simulink model "twin_sldemo_autotrans_old"  (Simulink 9.0)
settings: Solver=ode5  StartTime=0.0  StopTime=150.0  RelTol=1e-3  AbsTol=1e-6
model workspace (MAT data in the model file):
  CONVERTER_DATA = [0  137.465208994  2.232; 0.1  137.065019157  2.075; 0.2  135.864449646  1.975; 0.3  135.664354728  1.846; 0.4  137.565256453  1.72; 0.5  140.366585312  1.564; 0.6  145.268910814  1.409; 0.7  152.872517717  1.254; 0.8  162.9773111  1.096; 0.81  164.27792807  1.08; 0.82  166.178829795  1.061; 0.83  167.979684062  1.043; 0.84  170.080680706  1.028; 0.85  172.781962105  1.012; 0.86  175.383196045  1.002; 0.87  179.585189333  1.002; 0.88  183.587087703  1.001; 0.89  189.890077635  0.998; 0.9  197.693779455  0.999; 0.92  215.902417037  1.001; 0.94  244.515990379  1.002]
  DOWN_TABLE = [0  5  20  35; 0  5  20  35; 0  5  25  40; 0  5  30  50; 0  30  50  80; 0  30  50  80]
  DOWN_TH_BP = [0; 5; 40; 50; 90; 100]
  EMAP = [-40  -44  -49  -53  -57  -61  -65  -70  -74  -78  -82; 215  117  85  66  44  29  10  -2  -13  -22  -32; 245  208  178  148  122  104  85  66  48  33  18; 264  260  241  219  193  167  152  133  119  96  85; 264  279  282  275  260  238  223  208  189  171  152; 267  290  293  297  290  275  260  256  234  212  193; 267  297  305  305  305  301  293  282  267  249  226; 267  301  308  312  319  323  319  316  297  279  253; 267  301  312  319  327  327  327  327  312  293  267; 267  301  312  319  327  334  334  334  319  305  275]
  Iei = 0.0219914882836
  NE_VEC = [800 1200 1600 2000 2400 2800 3200 3600 4000 4400 4800]
  TH_VEC = [0; 20; 30; 40; 50; 60; 70; 80; 90; 100]
  TWAIT = 2
  UP_TABLE = [10  30  50  1000000; 10  30  50  1000000; 15  30  50  1000000; 23  41  60  1000000; 40  70  100  1000000; 40  70  100  1000000]
  UP_TH_BP = [0; 25; 35; 50; 90; 100]
  VEHICLE_DATA : num (value not decoded)
undefined symbols (not defined in the file or in its folder): sigbuilder_block
Description:
  | Modeling an Automatic Transmission Controller
  | 
  | In this example, Simulink(R) is used to model an automotive drivetrain. Stateflow(R)
  | enhances the Simulink model with its representation of the transmission
  | control logic. Simulink provides a powerful environment for the modeling and
  | simulation of dynamic systems and processes. In many systems, though,
  | supervisory functions like changing modes or invoking new gain schedules must
  | respond to events that may occur and conditions that develop over time. As a
  | result, the environment requires a language capable of managing these multiple
  | modes and developing conditions. In the following example, Stateflow
  | demonstrates its strength in this capacity by performing the function of gear
  | selection in an automatic transmission. This function is combined with the
  | drivetrain dynamics in a natural and intuitive manner by incorporating a
  | Stateflow block in the Simulink block diagram.
settings Model: SuppressorTable=22 serialization::archive 11 0 6 0 0 0 1 0  DataTypeOverride=Double  MinMaxOverflowLogging=ForceOff  FPTRunName=Active  Creator=The MathWorks, Inc.  LastModifiedBy=luigi  ExtModeTrigMode=oneshot  ExtModeArmWhenConnect=off  ExtModeAutoUpdateStatusClock=off
settings DataIOCC: SaveFormat=StructureWithTime  SaveOutput=off  SaveTime=off  SignalLoggingName=sldemo_autotrans_output
settings OptimizationCC: BlockReduction=off  ExpressionDepthLimit=2147483647  InitFltsAndDblsToZero=on
settings DebuggingCC: SignalInfNanChecking=error  SaveWithParameterizedLinksMsg=none  UnderspecifiedInitializationDetection=Simplified  MergeDetectMultiDrivingBlocksExec=error  CheckExecutionContextPreStartOutputMsg=on  CheckExecutionContextRuntimeOutputMsg=on  MultiTaskCondExecSysMsg=none  SigSpecEnsureSampleTimeMsg=none  IntegerOverflowMsg=none  FcnCallInpInsideContextMsg=warning  SignalLabelMismatchMsg=error  UnconnectedInputMsg=error  UnconnectedOutputMsg=error  UnconnectedLineMsg=error  UniqueDataStoreMsg=error  BusObjectLabelMismatch=error  RootOutportRequireBusObject=error  StateNameClashWarn=warning  StrictBusMsg=ErrorOnBusTreatedAsVector  NonBusSignalsTreatedAsBus=error  IntegerSaturationMsg=none
settings HardwareCC: ProdIntDivRoundTo=Floor
settings SFSimCC: SFSimEcho=off  SimParseCustomCode=off
settings GRTTargetCC: TargetFcnLib=ansi_tfl_tmw.mat  GeneratePreprocessorConditionals=Disable all  CombineOutputUpdateFcns=off  GRTInterface=on
settings ConfigComp: CovMetricSettings=dcmtr  CovHTMLOptions=-aTS=1 -bRG=1 -bTC=1 -hTR=0 -nFC=0 -scm=1 -bcm=1 -xEv=0  CovHtmlReporting=off

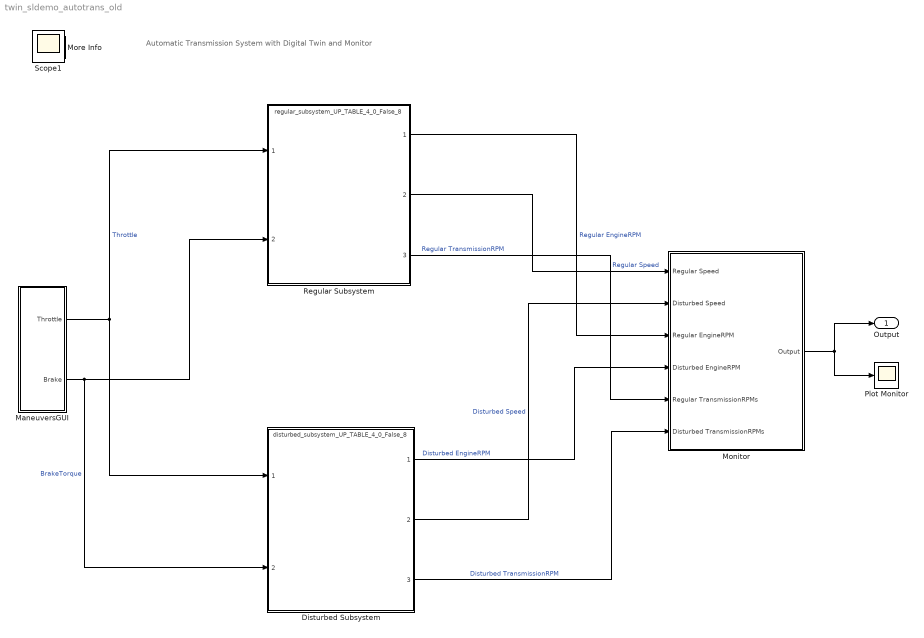
== system twin_sldemo_autotrans_old ==
  note: Automatic Transmission System with Digital Twin and Monitor
  Disturbed Subsystem : ModelReference  ModelNameDialog=disturbed_subsystem_UP_TABLE_4_0_False_8.mdl  SimulationMode=Normal  ModelReferenceVersion=1.265
  ManeuversGUI : Subsystem  Tag=STV Subsys  LoadFcn=sigbuilder_block('load');  StartFcn=sigbuilder_block('start');  StopFcn=sigbuilder_block('stop');  ClipboardFcn=sigbuilder_block('clipboard');  mask(Sigbuilder block){tuvar=[0:10]}
      mask help: Sigbuilder GUI
      mask init:
      | tuvar = sigbuilder_block('maskInit');
      settings: CopyFcn=sigbuilder_block('copy');  DeleteFcn=sigbuilder_block('delete');  ModelCloseFcn=sigbuilder_block('modelClose');  PreSaveFcn=sigbuilder_block('preSave');  PauseFcn=sigbuilder_block('pause')  ContinueFcn=sigbuilder_block('continue')  NameChangeFcn=sigbuilder_block('namechange');  OpenFcn=sigbuilder_block('open',[50.25 0 1389.75 726 ]);  CloseFcn=sigbuilder_block('close');
      mask Display: plot(0, 0, 100, 100,[2, 2, 32, 32, 2], [68, 8, 8, 68, 68],[32, 2], [38, 38], [32, 19, 2],[53, 60, 44], [32, 17, 17, 2],[16, 16, 31, 31]);txt = getActiveGroup(gcbh);text(2, 100, txt,'verticalAlignment', 'top');
  Monitor : Subsystem
  More Info : Subsystem
      settings: OpenFcn=showdemo(bdroot(gcb))
      mask Display: disp('?')
  Plot Monitor : Scope
  Regular Subsystem : ModelReference  ModelNameDialog=regular_subsystem_UP_TABLE_4_0_False_8.mdl  SimulationMode=Normal  ModelReferenceVersion=1.263
  Output : Outport
  Scope1 : Scope
  wires:
  Disturbed Subsystem/2 -> Monitor/2(Disturbed Speed)  "Disturbed Speed"
  ManeuversGUI/1(Throttle) -> Disturbed Subsystem/1, Regular Subsystem/1  "Throttle"
  Disturbed Subsystem/3 -> Monitor/6(Disturbed TransmissionRPMs)  "Disturbed TransmissionRPM"
  ManeuversGUI/2(Brake) -> Disturbed Subsystem/2, Regular Subsystem/2  "BrakeTorque"
  Monitor/1(Output) -> Plot Monitor/1, Output/1
  Regular Subsystem/1 -> Monitor/3(Regular EngineRPM)  "Regular EngineRPM"
  Regular Subsystem/2 -> Monitor/1(Regular Speed)  "Regular Speed"
  Regular Subsystem/3 -> Monitor/5(Regular TransmissionRPMs)  "Regular TransmissionRPM"
  Disturbed Subsystem/1 -> Monitor/4(Disturbed EngineRPM)  "Disturbed EngineRPM"

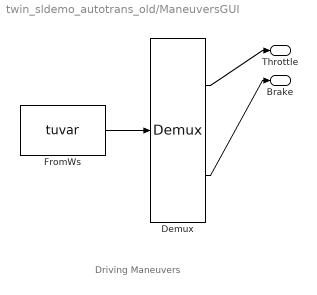
== system twin_sldemo_autotrans_old/ManeuversGUI ==
  note: Driving Maneuvers
  Demux : Demux  Tag=STV Demux  Outputs=2
  FromWs : FromWorkspace  Tag=STV FromWs  VariableName=tuvar  SampleTime=0  SigBuilderData=DataTag1  VnvData=DataTag2
      SigBuilderData=|
      | dataSet(1).timeRange = [0 150]
      | dataSet(1).name = 'Passing Maneuver'
      | dataSet(2).timeRange = [0 50]
      | dataSet(2).name = 'Gradual Acceleration'
      | dataSet(3).timeRange = [0 150]
      | dataSet(3).name = 'Hard braking'
      | dataSet(4).timeRange = [0 50]
      | dataSet(4).name = 'Coasting'
      | sbobj.Groups(1).Name = 'Passing Maneuver'
      | sbobj.Groups(1).Signals(1).Name = 'Throttle'
      | sbobj.Groups(1).Signals(1).XData = [0 150]
      | sbobj.Groups(1).Signals(1).YData = [100 100]
      | sbobj.Groups(1).Signals(2).Name = 'Brake'
      | sbobj.Groups(1).Signals(2).XData = [0 150]
      | sbobj.Groups(1).Signals(2).YData = [5650 5650]
      | sbobj.Groups(1).TimeRange = [0 150]
      | sbobj.Groups(2).Name = 'Gradual Acceleration'
      | sbobj.Groups(2).Signals(1).Name = 'Throttle'
      | sbobj.Groups(2).Signals(1).XData = [0 50]
      | sbobj.Groups(2).Signals(1).YData = [13.4 24]
      | sbobj.Groups(2).Signals(2).Name = 'Brake'
      | sbobj.Groups(2).Signals(2).XData = [0 50]
      | sbobj.Groups(2).Signals(2).YData = [0 0]
      | sbobj.Groups(2).TimeRange = [0 50]
      | sbobj.Groups(3).Name = 'Hard braking'
      | sbobj.Groups(3).Signals(1).Name = 'Throttle'
      | sbobj.Groups(3).Signals(1).XData = [0 5.1 150]
      | sbobj.Groups(3).Signals(1).YData = [100 100 100]
      | sbobj.Groups(3).Signals(2).Name = 'Brake'
      | sbobj.Groups(3).Signals(2).XData = [0 10 150]
      | sbobj.Groups(3).Signals(2).YData = [1150 1150 1150]
      | sbobj.Groups(3).TimeRange = [0 150]
      | sbobj.Groups(4).Name = 'Coasting'
      | sbobj.Groups(4).Signals(1).Name = 'Throttle'
      | sbobj.Groups(4).Signals(1).XData = [0 4.8 4.8 50]
      | sbobj.Groups(4).Signals(1).YData = [80 80 1 1]
      | sbobj.Groups(4).Signals(2).Name = 'Brake'
      | sbobj.Groups(4).Signals(2).XData = [0 50]
      | sbobj.Groups(4).Signals(2).YData = [0 0]
      | sbobj.Groups(4).TimeRange = [0 50]
  Throttle : Outport  Tag=STV Outport
  Brake : Outport  Tag=STV Outport  Port=2
  wires:
  FromWs/1 -> Demux/1
  Demux/1 -> Throttle/1
  Demux/2 -> Brake/1

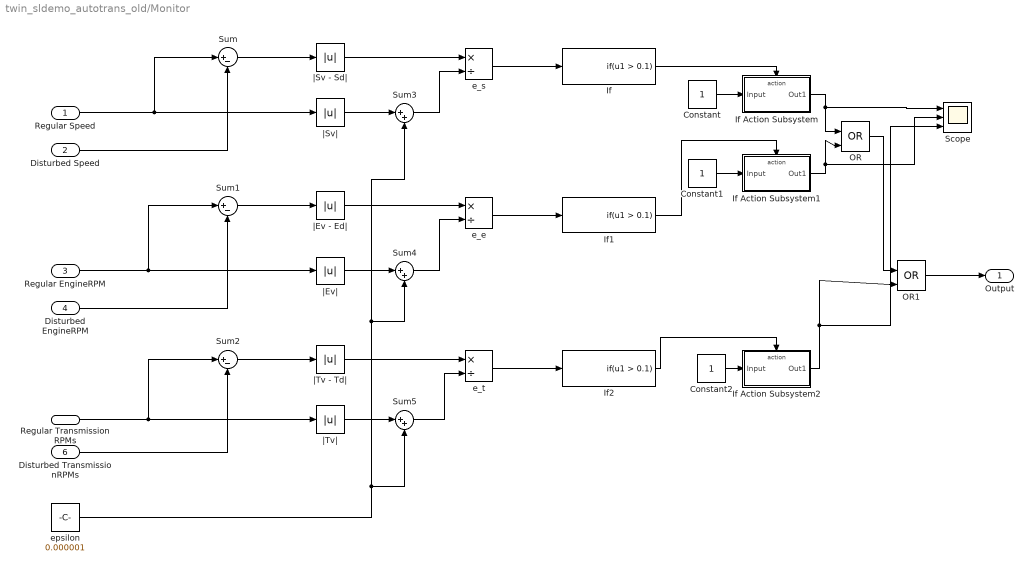
== system twin_sldemo_autotrans_old/Monitor ==
  Regular Speed : Inport
  Disturbed Speed : Inport  Port=2
  Regular EngineRPM : Inport  Port=3
  Disturbed EngineRPM : Inport  Port=4
  Regular TransmissionRPMs : Inport  Port=5
  Disturbed TransmissionRPMs : Inport  Port=6
  Constant : Constant
  Constant1 : Constant
  Constant2 : Constant
  If : If  IfExpression=u1 > 0.1  ShowElse=off
  If Action Subsystem : Subsystem  TreatAsAtomicUnit=on
  If Action Subsystem1 : Subsystem  TreatAsAtomicUnit=on
  If Action Subsystem2 : Subsystem  TreatAsAtomicUnit=on
  If1 : If  IfExpression=u1 > 0.1  ShowElse=off
  If2 : If  IfExpression=u1 > 0.1  ShowElse=off
  OR : Logic  Operator=OR  IconShape=distinctive  AllPortsSameDT=off  OutDataTypeStr=boolean
  OR1 : Logic  Operator=OR  IconShape=distinctive  AllPortsSameDT=off  OutDataTypeStr=boolean
  Scope : Scope  NumInputPorts=3
  Sum : Sum  Inputs=|+-
  Sum1 : Sum  Inputs=|+-
  Sum2 : Sum  Inputs=|+-
  Sum3 : Sum  Inputs=|++
  Sum4 : Sum  Inputs=|++
  Sum5 : Sum  Inputs=|++
  e_e : Product  Inputs=*/
  e_s : Product  Inputs=*/
  e_t : Product  Inputs=*/
  epsilon : Constant  Value=0.000001
  |Ev - Ed| : Abs
  |Ev| : Abs
  |Sv - Sd| : Abs
  |Sv| : Abs
  |Tv - Td| : Abs
  |Tv| : Abs
  Output : Outport
  wires:
  Regular Speed/1 -> Sum/1, |Sv|/1
  Disturbed Speed/1 -> Sum/2
  Regular EngineRPM/1 -> |Ev|/1, Sum1/1
  Disturbed EngineRPM/1 -> Sum1/2
  Regular TransmissionRPMs/1 -> Sum2/1, |Tv|/1
  Disturbed TransmissionRPMs/1 -> Sum2/2
  Sum/1 -> |Sv - Sd|/1
  Sum1/1 -> |Ev - Ed|/1
  Sum2/1 -> |Tv - Td|/1
  |Sv|/1 -> Sum3/1
  Sum3/1 -> e_s/2
  |Sv - Sd|/1 -> e_s/1
  e_s/1 -> If/1
  epsilon/1 -> Sum5/2, Sum4/2, Sum3/2
  |Tv|/1 -> Sum5/1
  |Ev|/1 -> Sum4/1
  |Ev - Ed|/1 -> e_e/1
  |Tv - Td|/1 -> e_t/1
  Sum5/1 -> e_t/2
  Sum4/1 -> e_e/2
  e_e/1 -> If1/1
  e_t/1 -> If2/1
  If1/1 -> If Action Subsystem1/Action
  OR/1 -> OR1/1
  If2/1 -> If Action Subsystem2/Action
  OR1/1 -> Output/1
  If/1 -> If Action Subsystem/Action
  If Action Subsystem/1(Out1) -> Scope/1, OR/1
  If Action Subsystem1/1(Out1) -> Scope/2, OR/2
  If Action Subsystem2/1(Out1) -> Scope/3, OR1/2
  Constant/1 -> If Action Subsystem/1(Input)
  Constant1/1 -> If Action Subsystem1/1(Input)
  Constant2/1 -> If Action Subsystem2/1(Input)

== system twin_sldemo_autotrans_old/More Info ==

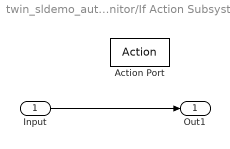
== system twin_sldemo_autotrans_old/Monitor/If Action Subsystem ==
  Input : Inport
  Action Port : ActionPort  ActionType=then
  Out1 : Outport
  wires:
  Input/1 -> Out1/1

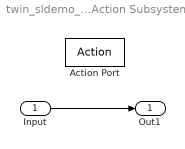
== system twin_sldemo_autotrans_old/Monitor/If Action Subsystem1 ==
  Input : Inport
  Action Port : ActionPort  ActionType=then
  Out1 : Outport
  wires:
  Input/1 -> Out1/1

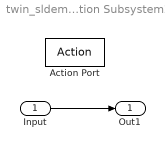
== system twin_sldemo_autotrans_old/Monitor/If Action Subsystem2 ==
  Input : Inport
  Action Port : ActionPort  ActionType=then
  Out1 : Outport
  wires:
  Input/1 -> Out1/1
